simulink model "Q_1"  (R2020a)
settings: Solver=VariableStepAuto  StartTime=0.0  StopTime=10.0  RelTol=1e-3
settings Model: EnablePacing=on  PacingRate=0.056000  Creator=Admin  LastModifiedBy=Admin

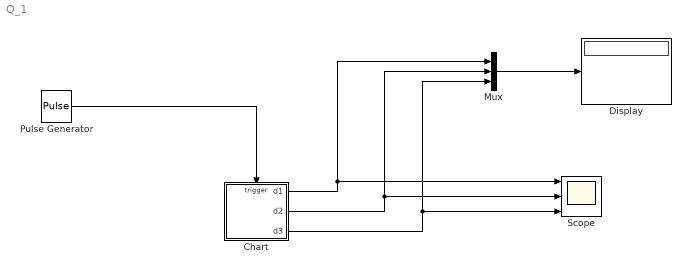
== system Q_1 ==
  Chart : Stateflow chart  TreatAsAtomicUnit=on
  Display : Display
  Mux : Mux  Inputs=3
  Pulse Generator : DiscretePulseGenerator  PulseType=Time based  Period=0.5  PulseWidth=5
  Scope : Scope  NumInputPorts=3
  wires:
  Mux/1 -> Display/1
  Chart/1(d1) -> Scope/1, Mux/1
  Chart/2(d2) -> Scope/2, Mux/2
  Chart/3(d3) -> Scope/3, Mux/3
  Pulse Generator/1 -> Chart/Trigger

== stateflow chart Q_1/Chart ==
  state digit1 [parallel]
    settings: executionOrder=1
    state one
      entry:
      d1=1;
    state zero
      entry:
      d1=0;
    state two
      entry:
      d1=2;
    state four
      entry:
      d1=4;
    state three
      entry:
      d1=3;
    digit1.one -> digit1.two : InputClick
    digit1.zero -> digit1.one : InputClick
    (default) -> digit1.zero
    digit1.four -> digit1.zero : InputClick{inc1}
    digit1.two -> digit1.three : InputClick
    digit1.three -> digit1.four : InputClick
  state digit2 [parallel]
    settings: executionOrder=2
    state one
      entry:
      d2=1;
    state zero
      entry:
      d2=0;
    state two
      entry:
      d2=2;
    state four
      entry:
      d2=4;
    state three
      entry:
      d2=3;
    digit2.one -> digit2.two : inc1
    digit2.zero -> digit2.one : inc1
    (default) -> digit2.zero
    digit2.four -> digit2.zero : inc1{inc2}
    digit2.two -> digit2.three : inc1
    digit2.three -> digit2.four : inc1
  state digit3 [parallel]
    settings: executionOrder=3
    state one
      entry:
      d3=1;
    state zero
      entry:
      d3=0;
    state two
      entry:
      d3=2;
    state four
      entry:
      d3=4;
    state three
      entry:
      d3=3;
    digit3.one -> digit3.two : inc2
    digit3.zero -> digit3.one : inc2
    (default) -> digit3.zero
    digit3.four -> digit3.zero : inc2
    digit3.two -> digit3.three : inc2
    digit3.three -> digit3.four : inc2
  data: d1 output; d2 output; d3 output
  events: InputClick input RISING_EDGE_EVENT; inc1 local RISING_EDGE_EVENT; inc2 local RISING_EDGE_EVENT
